simulink library "Memory_Blocks_Lib"  (Simulink 8.7)
settings: Solver=ode45  StartTime=0.0  StopTime=10.0  RelTol=1e-3
libraries: Memory_Blocks_Lib x72, simulink_extras x26, Decoders_Lib x7, Bit_Multiplexers_Lib x5, Byte_Multiplexers_Lib x2, Word_Multiplexers_Lib x1, commutil2 x1
(part 1 of 2)
settings Model: Creator=uzivatel  LastModifiedBy=Jozko Mrkvicka

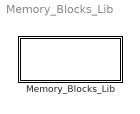
== system Memory_Blocks_Lib ==
  Memory_Blocks_Lib : Subsystem

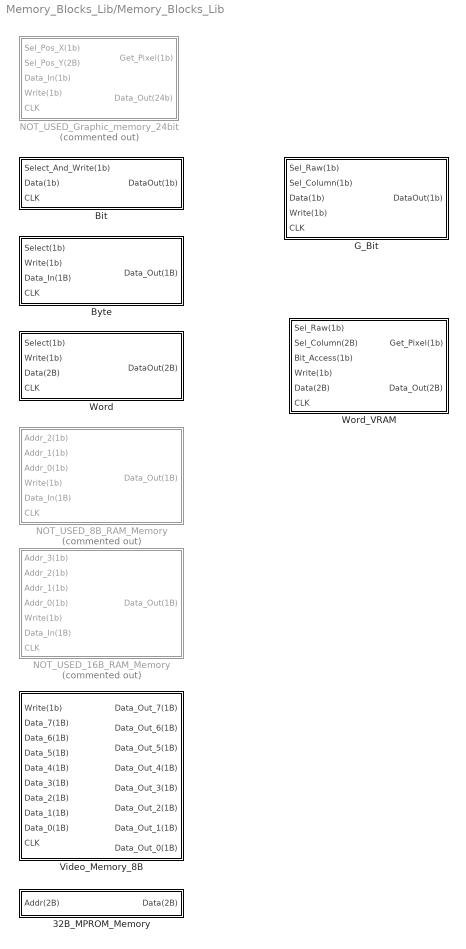
== system Memory_Blocks_Lib/Memory_Blocks_Lib ==
  32B_MPROM_Memory : Subsystem
  Bit : Subsystem
  Byte : Subsystem
  G_Bit : Subsystem
  NOT_USED_16B_RAM_Memory : Subsystem  Commented=on
  NOT_USED_8B_RAM_Memory : Subsystem  Commented=on
  NOT_USED_Graphic_memory_24bit : Subsystem  Commented=on
  Video_Memory_8B : Subsystem
  Word : Subsystem
  Word_VRAM : Subsystem

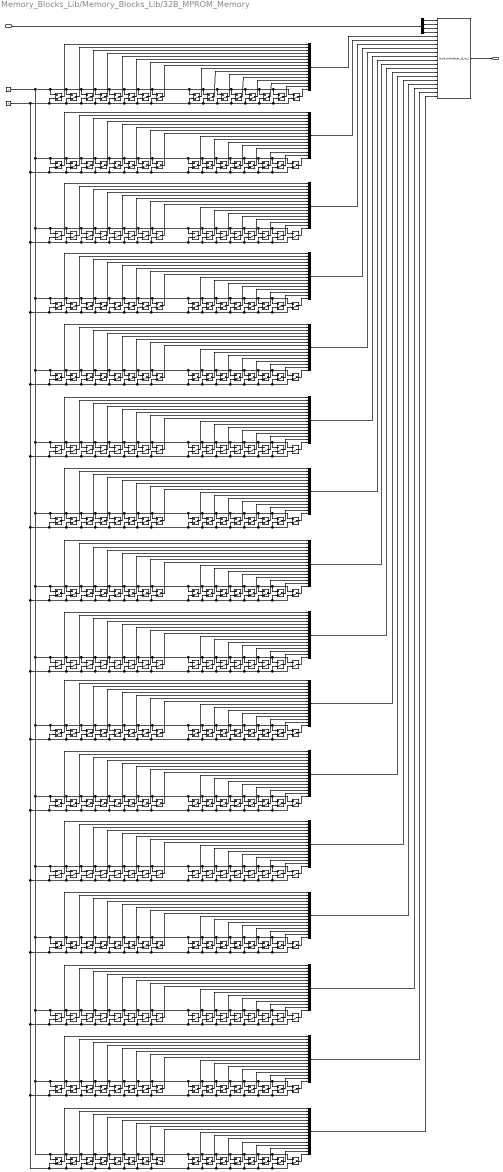
== system Memory_Blocks_Lib/Memory_Blocks_Lib/32B_MPROM_Memory ==
  note: Manually Programmable Read Only Memory (MPROM)
  Addr(2B) : Inport
  Bus Creator{,1..15} (16 alike) : BusCreator  Inputs=16
  Bus Selector : BusSelector  OutputSignals=signal13,signal14,signal15,signal16
  Constant : Constant
  Constant1 : Constant  Value=0
  Manual Switch{,1..156,158..255} (255 alike) : ManualSwitch  CurrentSetting=0
  Manual Switch157 : ManualSwitch
  Word_Multiplexer_16_to_1 : Word_Multiplexers_Lib/Word_Multiplexers_Lib/Word_Multiplexer_16_to_1
  Data(2B) : Outport
  wires:
  Addr(2B)/1 -> Bus Selector/1
  Manual Switch54/1 -> Bus Creator3/16
  Manual Switch59/1 -> Bus Creator3/7
  Manual Switch50/1 -> Bus Creator3/12
  Manual Switch57/1 -> Bus Creator3/5
  Manual Switch53/1 -> Bus Creator3/15
  Manual Switch48/1 -> Bus Creator3/1
  Manual Switch61/1 -> Bus Creator3/9
  Manual Switch52/1 -> Bus Creator3/14
  Manual Switch51/1 -> Bus Creator3/13
  Manual Switch56/1 -> Bus Creator3/4
  Manual Switch49/1 -> Bus Creator3/3
  Manual Switch58/1 -> Bus Creator3/6
  Manual Switch63/1 -> Bus Creator3/11
  Manual Switch62/1 -> Bus Creator3/10
  Manual Switch60/1 -> Bus Creator3/8
  Manual Switch55/1 -> Bus Creator3/2
  Manual Switch14/1 -> Bus Creator/16
  Manual Switch4/1 -> Bus Creator/6
  Manual Switch5/1 -> Bus Creator/7
  Manual Switch3/1 -> Bus Creator/5
  Manual Switch/1 -> Bus Creator/1
  Manual Switch99/1 -> Bus Creator6/13
  Manual Switch98/1 -> Bus Creator6/12
  Manual Switch111/1 -> Bus Creator6/11
  Manual Switch100/1 -> Bus Creator6/14
  Manual Switch110/1 -> Bus Creator6/10
  Manual Switch108/1 -> Bus Creator6/8
  Manual Switch109/1 -> Bus Creator6/9
  Manual Switch102/1 -> Bus Creator6/16
  Manual Switch101/1 -> Bus Creator6/15
  Manual Switch107/1 -> Bus Creator6/7
  Manual Switch104/1 -> Bus Creator6/4
  Manual Switch97/1 -> Bus Creator6/3
  Manual Switch103/1 -> Bus Creator6/2
  Manual Switch96/1 -> Bus Creator6/1
  Manual Switch105/1 -> Bus Creator6/5
  Manual Switch106/1 -> Bus Creator6/6
  Manual Switch85/1 -> Bus Creator5/15
  Manual Switch83/1 -> Bus Creator5/13
  Manual Switch82/1 -> Bus Creator5/12
  Manual Switch86/1 -> Bus Creator5/16
  Manual Switch84/1 -> Bus Creator5/14
  Manual Switch93/1 -> Bus Creator5/9
  Manual Switch91/1 -> Bus Creator5/7
  Manual Switch95/1 -> Bus Creator5/11
  Manual Switch94/1 -> Bus Creator5/10
  Manual Switch92/1 -> Bus Creator5/8
  Manual Switch90/1 -> Bus Creator5/6
  Manual Switch89/1 -> Bus Creator5/5
  Manual Switch88/1 -> Bus Creator5/4
  Manual Switch81/1 -> Bus Creator5/3
  Manual Switch87/1 -> Bus Creator5/2
  Manual Switch80/1 -> Bus Creator5/1
  Manual Switch130/1 -> Bus Creator8/12
  Manual Switch245/1 -> Bus Creator8/11
  Manual Switch234/1 -> Bus Creator8/10
  Manual Switch168/1 -> Bus Creator8/4
  Manual Switch141/1 -> Bus Creator8/13
  Manual Switch128/1 -> Bus Creator8/1
  Manual Switch169/1 -> Bus Creator9/14
  Manual Switch167/1 -> Bus Creator9/13
  Manual Switch166/1 -> Bus Creator9/12
  Manual Switch129/1 -> Bus Creator8/3
  Manual Switch170/1 -> Bus Creator9/15
  Manual Switch162/1 -> Bus Creator8/16
  Manual Switch161/1 -> Bus Creator8/15
  Manual Switch163/1 -> Bus Creator8/2
  Manual Switch171/1 -> Bus Creator9/16
  Manual Switch179/1 -> Bus Creator8/5
  Manual Switch223/1 -> Bus Creator8/9
  Manual Switch212/1 -> Bus Creator8/8
  Manual Switch201/1 -> Bus Creator8/7
  Manual Switch152/1 -> Bus Creator8/14
  Manual Switch190/1 -> Bus Creator8/6
  Manual Switch186/1 -> Bus Creator10/14
  Manual Switch184/1 -> Bus Creator10/12
  Manual Switch197/1 -> Bus Creator10/10
  Manual Switch192/1 -> Bus Creator10/5
  Manual Switch211/1 -> Bus Creator11/7
  Manual Switch209/1 -> Bus Creator11/5
  Manual Switch187/1 -> Bus Creator10/15
  Manual Switch173/1 -> Bus Creator9/4
  Manual Switch195/1 -> Bus Creator10/8
  Manual Switch200/1 -> Bus Creator11/3
  Manual Switch216/1 -> Bus Creator11/11
  Manual Switch199/1 -> Bus Creator11/1
  Manual Switch178/1 -> Bus Creator9/9
  Manual Switch191/1 -> Bus Creator10/4
  Manual Switch214/1 -> Bus Creator11/9
  Manual Switch221/1 -> Bus Creator12/14
  Manual Switch220/1 -> Bus Creator12/13
  Manual Switch232/1 -> Bus Creator12/10
  Manual Switch213/1 -> Bus Creator11/8
  Manual Switch233/1 -> Bus Creator12/11
  Manual Switch231/1 -> Bus Creator12/9
  Manual Switch174/1 -> Bus Creator9/5
  Manual Switch177/1 -> Bus Creator9/8
  Manual Switch189/1 -> Bus Creator10/2
  Manual Switch180/1 -> Bus Creator9/10
  Manual Switch182/1 -> Bus Creator10/1
  Manual Switch203/1 -> Bus Creator11/13
  Manual Switch204/1 -> Bus Creator11/14
  Manual Switch205/1 -> Bus Creator11/15
  Manual Switch181/1 -> Bus Creator9/11
  Manual Switch196/1 -> Bus Creator10/9
  Manual Switch207/1 -> Bus Creator11/2
  Manual Switch222/1 -> Bus Creator12/15
  Manual Switch219/1 -> Bus Creator12/12
  Manual Switch230/1 -> Bus Creator12/8
  Manual Switch198/1 -> Bus Creator10/11
  Manual Switch183/1 -> Bus Creator10/3
  Manual Switch208/1 -> Bus Creator11/4
  Manual Switch194/1 -> Bus Creator10/7
  Manual Switch165/1 -> Bus Creator9/3
  Manual Switch172/1 -> Bus Creator9/2
  Manual Switch229/1 -> Bus Creator12/7
  Manual Switch228/1 -> Bus Creator12/6
  Manual Switch227/1 -> Bus Creator12/5
  Manual Switch202/1 -> Bus Creator11/12
  Manual Switch175/1 -> Bus Creator9/6
  Manual Switch185/1 -> Bus Creator10/13
  Manual Switch215/1 -> Bus Creator11/10
  Manual Switch164/1 -> Bus Creator9/1
  Manual Switch188/1 -> Bus Creator10/16
  Manual Switch210/1 -> Bus Creator11/6
  Manual Switch193/1 -> Bus Creator10/6
  Manual Switch224/1 -> Bus Creator12/16
  Manual Switch206/1 -> Bus Creator11/16
  Manual Switch176/1 -> Bus Creator9/7
  Manual Switch143/1 -> Bus Creator14/11
  Manual Switch236/1 -> Bus Creator13/3
  Manual Switch153/1 -> Bus Creator15/4
  Manual Switch132/1 -> Bus Creator14/15
  Manual Switch140/1 -> Bus Creator14/9
  Manual Switch252/1 -> Bus Creator14/1
  Manual Switch240/1 -> Bus Creator13/15
  Constant/1 -> Manual Switch17/1, Manual Switch24/1, Manual Switch22/1, Manual Switch21/1, Manual Switch20/1, Manual Switch19/1, Manual Switch18/1, Manual Switch31/1, Manual Switch30/1, Manual Switch29/1, Manual Switch28/1, Manual Switch27/1, Manual Switch26/1, Manual Switch25/1, Manual Switch23/1, Manual Switch16/1, Manual Switch33/1, Manual Switch40/1, Manual Switch38/1, Manual Switch37/1, Manual Switch36/1, Manual Switch35/1, Manual Switch34/1, Manual Switch47/1, Manual Switch46/1, Manual Switch45/1, Manual Switch44/1, Manual Switch43/1, Manual Switch42/1, Manual Switch41/1, Manual Switch39/1, Manual Switch32/1, Manual Switch49/1, Manual Switch56/1, Manual Switch54/1, Manual Switch53/1, Manual Switch52/1, Manual Switch51/1, Manual Switch50/1, Manual Switch63/1, Manual Switch62/1, Manual Switch61/1, Manual Switch60/1, Manual Switch59/1, Manual Switch58/1, Manual Switch57/1, Manual Switch55/1, Manual Switch48/1, Manual Switch65/1, Manual Switch72/1, Manual Switch70/1, Manual Switch69/1, Manual Switch68/1, Manual Switch67/1, Manual Switch66/1, Manual Switch79/1, Manual Switch78/1, Manual Switch77/1, Manual Switch76/1, Manual Switch75/1, Manual Switch74/1, Manual Switch73/1, Manual Switch71/1, Manual Switch64/1, Manual Switch81/1, Manual Switch88/1, Manual Switch86/1, Manual Switch85/1, Manual Switch84/1, Manual Switch83/1, Manual Switch82/1, Manual Switch95/1, Manual Switch94/1, Manual Switch93/1, Manual Switch92/1, Manual Switch91/1, Manual Switch90/1, Manual Switch89/1, Manual Switch87/1, Manual Switch80/1, Manual Switch97/1, Manual Switch104/1, Manual Switch102/1, Manual Switch101/1, Manual Switch100/1, Manual Switch99/1, Manual Switch98/1, Manual Switch111/1, Manual Switch110/1, Manual Switch109/1, Manual Switch108/1, Manual Switch107/1, Manual Switch106/1, Manual Switch105/1, Manual Switch103/1, Manual Switch96/1, Manual Switch113/1, Manual Switch120/1, Manual Switch118/1, Manual Switch117/1, Manual Switch116/1, Manual Switch115/1, Manual Switch114/1, Manual Switch127/1, Manual Switch126/1, Manual Switch125/1, Manual Switch124/1, Manual Switch123/1, Manual Switch122/1, Manual Switch121/1, Manual Switch119/1, Manual Switch112/1, Manual Switch129/1, Manual Switch168/1, Manual Switch162/1, Manual Switch161/1, Manual Switch152/1, Manual Switch141/1, Manual Switch130/1, Manual Switch245/1, Manual Switch234/1, Manual Switch223/1, Manual Switch212/1, Manual Switch201/1, Manual Switch190/1, Manual Switch179/1, Manual Switch163/1, Manual Switch128/1, Manual Switch165/1, Manual Switch173/1, Manual Switch171/1, Manual Switch170/1, Manual Switch169/1, Manual Switch167/1, Manual Switch166/1, Manual Switch181/1, Manual Switch180/1, Manual Switch178/1, Manual Switch177/1, Manual Switch176/1, Manual Switch175/1, Manual Switch174/1, Manual Switch172/1, Manual Switch164/1, Manual Switch183/1, Manual Switch191/1, Manual Switch188/1, Manual Switch187/1, Manual Switch186/1, Manual Switch185/1, Manual Switch184/1, Manual Switch198/1, Manual Switch197/1, Manual Switch196/1, Manual Switch195/1, Manual Switch194/1, Manual Switch193/1, Manual Switch192/1, Manual Switch189/1, Manual Switch182/1, Manual Switch200/1, Manual Switch208/1, Manual Switch206/1, Manual Switch205/1, Manual Switch204/1, Manual Switch203/1, Manual Switch202/1, Manual Switch216/1, Manual Switch215/1, Manual Switch214/1, Manual Switch213/1, Manual Switch211/1, Manual Switch210/1, Manual Switch209/1, Manual Switch207/1, Manual Switch199/1, Manual Switch218/1, Manual Switch226/1, Manual Switch224/1, Manual Switch222/1, Manual Switch221/1, Manual Switch220/1, Manual Switch219/1, Manual Switch233/1, Manual Switch232/1, Manual Switch231/1, Manual Switch230/1, Manual Switch229/1, Manual Switch228/1, Manual Switch227/1, Manual Switch225/1, Manual Switch217/1, Manual Switch236/1, Manual Switch243/1, Manual Switch241/1, Manual Switch240/1, Manual Switch239/1, Manual Switch238/1, Manual Switch237/1, Manual Switch251/1, Manual Switch250/1, Manual Switch249/1, Manual Switch248/1, Manual Switch247/1, Manual Switch246/1, Manual Switch244/1, Manual Switch242/1, Manual Switch235/1, Manual Switch253/1, Manual Switch135/1, Manual Switch133/1, Manual Switch132/1, Manual Switch131/1, Manual Switch255/1, Manual Switch254/1, Manual Switch143/1, Manual Switch142/1, Manual Switch140/1, Manual Switch139/1, Manual Switch138/1, Manual Switch137/1, Manual Switch136/1, Manual Switch134/1, Manual Switch252/1, Manual Switch145/1, Manual Switch153/1, Manual Switch150/1, Manual Switch149/1, Manual Switch148/1, Manual Switch147/1, Manual Switch146/1, Manual Switch160/1, Manual Switch159/1, Manual Switch158/1, Manual Switch157/1, Manual Switch156/1, Manual Switch155/1, Manual Switch154/1, Manual Switch151/1, Manual Switch144/1, Manual Switch1/1, Manual Switch2/1, Manual Switch14/1, Manual Switch13/1, Manual Switch12/1, Manual Switch11/1, Manual Switch10/1, Manual Switch9/1, Manual Switch8/1, Manual Switch7/1, Manual Switch6/1, Manual Switch5/1, Manual Switch4/1, Manual Switch3/1, Manual Switch15/1, Manual Switch/1
  Manual Switch254/1 -> Bus Creator14/12
  Manual Switch159/1 -> Bus Creator15/10
  Manual Switch145/1 -> Bus Creator15/3
  Manual Switch151/1 -> Bus Creator15/2
  Manual Switch144/1 -> Bus Creator15/1
  Manual Switch139/1 -> Bus Creator14/8
  Manual Switch138/1 -> Bus Creator14/7
  Manual Switch134/1 -> Bus Creator14/2
  Manual Switch242/1 -> Bus Creator13/2
  Manual Switch239/1 -> Bus Creator13/14
  Manual Switch253/1 -> Bus Creator14/3
  Manual Switch251/1 -> Bus Creator13/11
  Manual Switch149/1 -> Bus Creator15/15
  Manual Switch217/1 -> Bus Creator12/1
  Manual Switch255/1 -> Bus Creator14/13
  Manual Switch249/1 -> Bus Creator13/9
  Manual Switch235/1 -> Bus Creator13/1
  Manual Switch131/1 -> Bus Creator14/14
  Manual Switch225/1 -> Bus Creator12/2
  Manual Switch218/1 -> Bus Creator12/3
  Manual Switch248/1 -> Bus Creator13/8
  Manual Switch136/1 -> Bus Creator14/5
  Manual Switch135/1 -> Bus Creator14/4
  Manual Switch147/1 -> Bus Creator15/13
  Manual Switch146/1 -> Bus Creator15/12
  Manual Switch237/1 -> Bus Creator13/12
  Manual Switch243/1 -> Bus Creator13/4
  Manual Switch250/1 -> Bus Creator13/10
  Manual Switch142/1 -> Bus Creator14/10
  Manual Switch148/1 -> Bus Creator15/14
  Manual Switch160/1 -> Bus Creator15/11
  Manual Switch238/1 -> Bus Creator13/13
  Manual Switch137/1 -> Bus Creator14/6
  Manual Switch158/1 -> Bus Creator15/9
  Manual Switch246/1 -> Bus Creator13/6
  Manual Switch247/1 -> Bus Creator13/7
  Manual Switch157/1 -> Bus Creator15/8
  Manual Switch244/1 -> Bus Creator13/5
  Manual Switch133/1 -> Bus Creator14/16
  Manual Switch150/1 -> Bus Creator15/16
  Manual Switch156/1 -> Bus Creator15/7
  Manual Switch155/1 -> Bus Creator15/6
  Manual Switch154/1 -> Bus Creator15/5
  Manual Switch226/1 -> Bus Creator12/4
  Manual Switch241/1 -> Bus Creator13/16
  Manual Switch13/1 -> Bus Creator/15
  Manual Switch6/1 -> Bus Creator/8
  Manual Switch11/1 -> Bus Creator/13
  Manual Switch9/1 -> Bus Creator/11
  Manual Switch15/1 -> Bus Creator/2
  Manual Switch8/1 -> Bus Creator/10
  Manual Switch10/1 -> Bus Creator/12
  Manual Switch33/1 -> Bus Creator2/3
  Manual Switch35/1 -> Bus Creator2/13
  Manual Switch44/1 -> Bus Creator2/8
  Manual Switch40/1 -> Bus Creator2/4
  Manual Switch43/1 -> Bus Creator2/7
  Manual Switch39/1 -> Bus Creator2/2
  Manual Switch36/1 -> Bus Creator2/14
  Manual Switch47/1 -> Bus Creator2/11
  Manual Switch41/1 -> Bus Creator2/5
  Manual Switch38/1 -> Bus Creator2/16
  Manual Switch34/1 -> Bus Creator2/12
  Manual Switch45/1 -> Bus Creator2/9
  Manual Switch32/1 -> Bus Creator2/1
  Manual Switch42/1 -> Bus Creator2/6
  Manual Switch46/1 -> Bus Creator2/10
  Manual Switch37/1 -> Bus Creator2/15
  Bus Creator2/1 -> Word_Multiplexer_16_to_1/7
  Bus Creator1/1 -> Word_Multiplexer_16_to_1/6
  Bus Creator5/1 -> Word_Multiplexer_16_to_1/10
  Bus Selector/1 -> Word_Multiplexer_16_to_1/1  "<signal13>"
  Bus Creator15/1 -> Word_Multiplexer_16_to_1/20
  Bus Selector/4 -> Word_Multiplexer_16_to_1/4  "<signal16>"
  Bus Creator11/1 -> Word_Multiplexer_16_to_1/16
  Bus Creator14/1 -> Word_Multiplexer_16_to_1/19
  Bus Creator/1 -> Word_Multiplexer_16_to_1/5
  Bus Creator9/1 -> Word_Multiplexer_16_to_1/14
  Bus Creator12/1 -> Word_Multiplexer_16_to_1/17
  Bus Creator13/1 -> Word_Multiplexer_16_to_1/18
  Bus Selector/2 -> Word_Multiplexer_16_to_1/2  "<signal14>"
  Bus Creator4/1 -> Word_Multiplexer_16_to_1/9
  Bus Creator6/1 -> Word_Multiplexer_16_to_1/11
  Bus Selector/3 -> Word_Multiplexer_16_to_1/3  "<signal15>"
  Bus Creator3/1 -> Word_Multiplexer_16_to_1/8
  Bus Creator8/1 -> Word_Multiplexer_16_to_1/13
  Bus Creator10/1 -> Word_Multiplexer_16_to_1/15
  Word_Multiplexer_16_to_1/1 -> Data(2B)/1
  Bus Creator7/1 -> Word_Multiplexer_16_to_1/12
  Manual Switch70/1 -> Bus Creator4/16
  Manual Switch69/1 -> Bus Creator4/15
  Manual Switch79/1 -> Bus Creator4/11
  Manual Switch75/1 -> Bus Creator4/7
  Manual Switch73/1 -> Bus Creator4/5
  Manual Switch68/1 -> Bus Creator4/14
  Manual Switch65/1 -> Bus Creator4/3
  Manual Switch71/1 -> Bus Creator4/2
  Manual Switch74/1 -> Bus Creator4/6
  Manual Switch76/1 -> Bus Creator4/8
  Manual Switch64/1 -> Bus Creator4/1
  Manual Switch72/1 -> Bus Creator4/4
  Manual Switch78/1 -> Bus Creator4/10
  Manual Switch66/1 -> Bus Creator4/12
  Manual Switch77/1 -> Bus Creator4/9
  Manual Switch67/1 -> Bus Creator4/13
  Manual Switch127/1 -> Bus Creator7/11
  Manual Switch125/1 -> Bus Creator7/9
  Manual Switch119/1 -> Bus Creator7/2
  Manual Switch122/1 -> Bus Creator7/6
  Manual Switch112/1 -> Bus Creator7/1
  Manual Switch121/1 -> Bus Creator7/5
  Manual Switch120/1 -> Bus Creator7/4
  Manual Switch113/1 -> Bus Creator7/3
  Manual Switch124/1 -> Bus Creator7/8
  Manual Switch126/1 -> Bus Creator7/10
  Manual Switch123/1 -> Bus Creator7/7
  Manual Switch2/1 -> Bus Creator/4
  Manual Switch12/1 -> Bus Creator/14
  Manual Switch115/1 -> Bus Creator7/13
  Manual Switch114/1 -> Bus Creator7/12
  Manual Switch7/1 -> Bus Creator/9
  Manual Switch1/1 -> Bus Creator/3
  Manual Switch118/1 -> Bus Creator7/16
  Manual Switch116/1 -> Bus Creator7/14
  Manual Switch117/1 -> Bus Creator7/15
  Manual Switch24/1 -> Bus Creator1/4
  Manual Switch22/1 -> Bus Creator1/16
  Manual Switch30/1 -> Bus Creator1/10
  Manual Switch26/1 -> Bus Creator1/6
  Manual Switch20/1 -> Bus Creator1/14
  Manual Switch19/1 -> Bus Creator1/13
  Constant1/1 -> Manual Switch23/2, Manual Switch17/2, Manual Switch25/2, Manual Switch26/2, Manual Switch22/2, Manual Switch21/2, Manual Switch20/2, Manual Switch19/2, Manual Switch18/2, Manual Switch31/2, Manual Switch30/2, Manual Switch29/2, Manual Switch28/2, Manual Switch27/2, Manual Switch24/2, Manual Switch16/2, Manual Switch39/2, Manual Switch33/2, Manual Switch41/2, Manual Switch42/2, Manual Switch38/2, Manual Switch37/2, Manual Switch36/2, Manual Switch35/2, Manual Switch34/2, Manual Switch47/2, Manual Switch46/2, Manual Switch45/2, Manual Switch44/2, Manual Switch43/2, Manual Switch40/2, Manual Switch32/2, Manual Switch55/2, Manual Switch49/2, Manual Switch57/2, Manual Switch58/2, Manual Switch54/2, Manual Switch53/2, Manual Switch52/2, Manual Switch51/2, Manual Switch50/2, Manual Switch63/2, Manual Switch62/2, Manual Switch61/2, Manual Switch60/2, Manual Switch59/2, Manual Switch56/2, Manual Switch48/2, Manual Switch71/2, Manual Switch65/2, Manual Switch73/2, Manual Switch74/2, Manual Switch70/2, Manual Switch69/2, Manual Switch68/2, Manual Switch67/2, Manual Switch66/2, Manual Switch79/2, Manual Switch78/2, Manual Switch77/2, Manual Switch76/2, Manual Switch75/2, Manual Switch72/2, Manual Switch64/2, Manual Switch103/2, Manual Switch97/2, Manual Switch105/2, Manual Switch106/2, Manual Switch102/2, Manual Switch101/2, Manual Switch100/2, Manual Switch99/2, Manual Switch98/2, Manual Switch111/2, Manual Switch110/2, Manual Switch109/2, Manual Switch108/2, Manual Switch107/2, Manual Switch104/2, Manual Switch96/2, Manual Switch119/2, Manual Switch113/2, Manual Switch121/2, Manual Switch122/2, Manual Switch118/2, Manual Switch117/2, Manual Switch116/2, Manual Switch115/2, Manual Switch114/2, Manual Switch127/2, Manual Switch126/2, Manual Switch125/2, Manual Switch124/2, Manual Switch123/2, Manual Switch120/2, Manual Switch112/2, Manual Switch163/2, Manual Switch129/2, Manual Switch179/2, Manual Switch190/2, Manual Switch162/2, Manual Switch161/2, Manual Switch152/2, Manual Switch141/2, Manual Switch130/2, Manual Switch245/2, Manual Switch234/2, Manual Switch223/2, Manual Switch212/2, Manual Switch201/2, Manual Switch168/2, Manual Switch128/2, Manual Switch172/2, Manual Switch165/2, Manual Switch174/2, Manual Switch175/2, Manual Switch171/2, Manual Switch170/2, Manual Switch169/2, Manual Switch167/2, Manual Switch166/2, Manual Switch181/2, Manual Switch180/2, Manual Switch178/2, Manual Switch177/2, Manual Switch176/2, Manual Switch173/2, Manual Switch164/2, Manual Switch189/2, Manual Switch183/2, Manual Switch192/2, Manual Switch193/2, Manual Switch188/2, Manual Switch187/2, Manual Switch186/2, Manual Switch185/2, Manual Switch184/2, Manual Switch198/2, Manual Switch197/2, Manual Switch196/2, Manual Switch195/2, Manual Switch194/2, Manual Switch191/2, Manual Switch182/2, Manual Switch207/2, Manual Switch200/2, Manual Switch209/2, Manual Switch210/2, Manual Switch206/2, Manual Switch205/2, Manual Switch204/2, Manual Switch203/2, Manual Switch202/2, Manual Switch216/2, Manual Switch215/2, Manual Switch214/2, Manual Switch213/2, Manual Switch211/2, Manual Switch208/2, Manual Switch199/2, Manual Switch225/2, Manual Switch218/2, Manual Switch227/2, Manual Switch228/2, Manual Switch224/2, Manual Switch222/2, Manual Switch221/2, Manual Switch220/2, Manual Switch219/2, Manual Switch233/2, Manual Switch232/2, Manual Switch231/2, Manual Switch230/2, Manual Switch229/2, Manual Switch226/2, Manual Switch217/2, Manual Switch242/2, Manual Switch236/2, Manual Switch244/2, Manual Switch246/2, Manual Switch241/2, Manual Switch240/2, Manual Switch239/2, Manual Switch238/2, Manual Switch237/2, Manual Switch251/2, Manual Switch250/2, Manual Switch249/2, Manual Switch248/2, Manual Switch247/2, Manual Switch243/2, Manual Switch235/2, Manual Switch134/2, Manual Switch253/2, Manual Switch136/2, Manual Switch137/2, Manual Switch133/2, Manual Switch132/2, Manual Switch131/2, Manual Switch255/2, Manual Switch254/2, Manual Switch143/2, Manual Switch142/2, Manual Switch140/2, Manual Switch139/2, Manual Switch138/2, Manual Switch135/2, Manual Switch252/2, Manual Switch151/2, Manual Switch145/2, Manual Switch154/2, Manual Switch155/2, Manual Switch150/2, Manual Switch149/2, Manual Switch148/2, Manual Switch147/2, Manual Switch146/2, Manual Switch160/2, Manual Switch159/2, Manual Switch158/2, Manual Switch157/2, Manual Switch156/2, Manual Switch153/2, Manual Switch144/2, Manual Switch87/2, Manual Switch81/2, Manual Switch89/2, Manual Switch90/2, Manual Switch86/2, Manual Switch85/2, Manual Switch84/2, Manual Switch83/2, Manual Switch82/2, Manual Switch95/2, Manual Switch94/2, Manual Switch93/2, Manual Switch92/2, Manual Switch91/2, Manual Switch88/2, Manual Switch80/2, Manual Switch15/2, Manual Switch1/2, Manual Switch3/2, Manual Switch4/2, Manual Switch14/2, Manual Switch13/2, Manual Switch12/2, Manual Switch11/2, Manual Switch10/2, Manual Switch9/2, Manual Switch8/2, Manual Switch7/2, Manual Switch6/2, Manual Switch5/2, Manual Switch2/2, Manual Switch/2
  Manual Switch27/1 -> Bus Creator1/7
  Manual Switch21/1 -> Bus Creator1/15
  Manual Switch25/1 -> Bus Creator1/5
  Manual Switch17/1 -> Bus Creator1/3
  Manual Switch31/1 -> Bus Creator1/11
  Manual Switch29/1 -> Bus Creator1/9
  Manual Switch28/1 -> Bus Creator1/8
  Manual Switch23/1 -> Bus Creator1/2
  Manual Switch16/1 -> Bus Creator1/1
  Manual Switch18/1 -> Bus Creator1/12

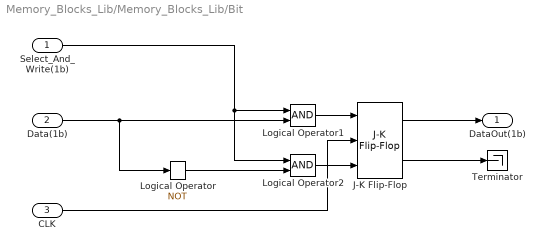
== system Memory_Blocks_Lib/Memory_Blocks_Lib/Bit ==
  Select_And_Write(1b) : Inport  OutDataTypeStr=boolean
  Data(1b) : Inport  Port=2  OutDataTypeStr=boolean
  CLK : Inport  Port=3  OutDataTypeStr=double
  J-K Flip-Flop : simulink_extras/Flip Flops/J-K Flip-Flop  initial_condition=0
  Logical Operator : Logic  Operator=NOT  IconShape=distinctive  AllPortsSameDT=off  OutDataTypeStr=boolean
  Logical Operator1 : Logic  IconShape=distinctive  AllPortsSameDT=off  OutDataTypeStr=boolean
  Logical Operator2 : Logic  IconShape=distinctive  AllPortsSameDT=off  OutDataTypeStr=boolean
  Terminator : Terminator
  DataOut(1b) : Outport
  wires:
  Data(1b)/1 -> Logical Operator/1, Logical Operator1/2
  J-K Flip-Flop/2 -> Terminator/1
  J-K Flip-Flop/1 -> DataOut(1b)/1
  CLK/1 -> J-K Flip-Flop/2
  Select_And_Write(1b)/1 -> Logical Operator2/1, Logical Operator1/1
  Logical Operator/1 -> Logical Operator2/2
  Logical Operator1/1 -> J-K Flip-Flop/1
  Logical Operator2/1 -> J-K Flip-Flop/3

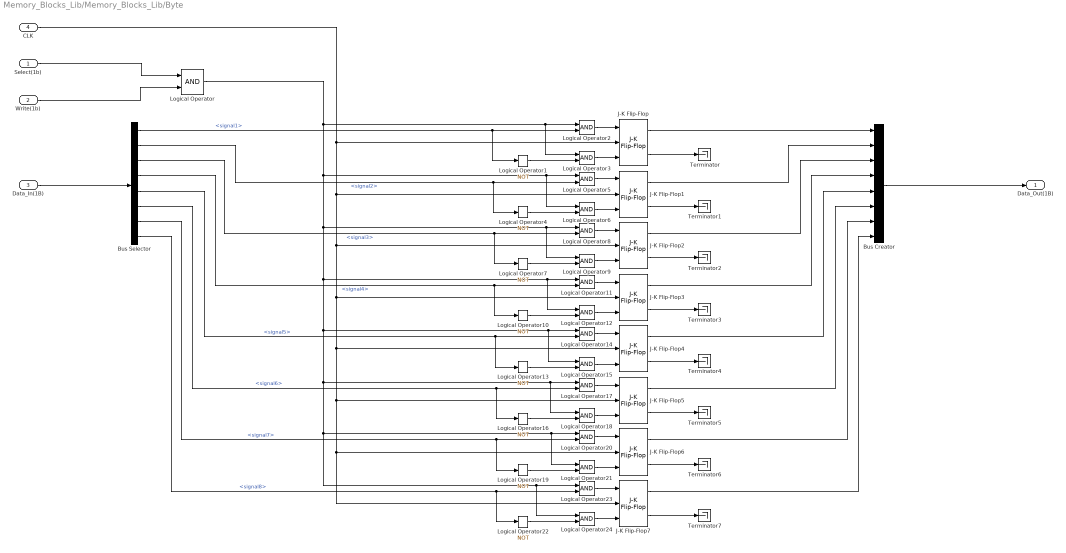
== system Memory_Blocks_Lib/Memory_Blocks_Lib/Byte ==
  Select(1b) : Inport
  Write(1b) : Inport  Port=2
  Data_In(1B) : Inport  Port=3
  CLK : Inport  Port=4  OutDataTypeStr=double
  Bus Creator : BusCreator  Inputs=8
  Bus Selector : BusSelector  OutputSignals=signal1,signal2,signal3,signal4,signal5,signal6,signal7,signal8
  J-K Flip-Flop{,1..7} (8 alike) : simulink_extras/Flip Flops/J-K Flip-Flop  initial_condition=0
  Logical Operator{,2..3,5..6,8..9,11..12,14..15,17..18,20..21,23..24} (17 alike) : Logic  IconShape=distinctive  AllPortsSameDT=off  OutDataTypeStr=boolean
  Logical Operator{1,4,7,10,13,16,19,22} (8 alike) : Logic  Operator=NOT  IconShape=distinctive  AllPortsSameDT=off  OutDataTypeStr=boolean
  Terminator{,1..7} (8 alike) : Terminator
  Data_Out(1B) : Outport
  wires:
  Write(1b)/1 -> Logical Operator/2
  Select(1b)/1 -> Logical Operator/1
  Data_In(1B)/1 -> Bus Selector/1
  J-K Flip-Flop7/1 -> Bus Creator/8
  J-K Flip-Flop6/1 -> Bus Creator/7
  J-K Flip-Flop5/1 -> Bus Creator/6
  J-K Flip-Flop4/1 -> Bus Creator/5
  J-K Flip-Flop3/1 -> Bus Creator/4
  J-K Flip-Flop2/1 -> Bus Creator/3
  J-K Flip-Flop1/1 -> Bus Creator/2
  J-K Flip-Flop/1 -> Bus Creator/1
  Bus Selector/1 -> Logical Operator1/1, Logical Operator2/2  "<signal1>"
  J-K Flip-Flop/2 -> Terminator/1
  Logical Operator1/1 -> Logical Operator3/2
  Logical Operator2/1 -> J-K Flip-Flop/1
  Logical Operator3/1 -> J-K Flip-Flop/3
  Bus Selector/2 -> Logical Operator4/1, Logical Operator5/2  "<signal2>"
  J-K Flip-Flop1/2 -> Terminator1/1
  Logical Operator4/1 -> Logical Operator6/2
  Logical Operator5/1 -> J-K Flip-Flop1/1
  Logical Operator6/1 -> J-K Flip-Flop1/3
  Bus Selector/3 -> Logical Operator7/1, Logical Operator8/2  "<signal3>"
  J-K Flip-Flop2/2 -> Terminator2/1
  Logical Operator7/1 -> Logical Operator9/2
  Logical Operator8/1 -> J-K Flip-Flop2/1
  Logical Operator9/1 -> J-K Flip-Flop2/3
  Bus Selector/4 -> Logical Operator11/2, Logical Operator10/1  "<signal4>"
  J-K Flip-Flop3/2 -> Terminator3/1
  Logical Operator10/1 -> Logical Operator12/2
  Logical Operator11/1 -> J-K Flip-Flop3/1
  Logical Operator12/1 -> J-K Flip-Flop3/3
  Bus Selector/5 -> Logical Operator14/2, Logical Operator13/1  "<signal5>"
  J-K Flip-Flop4/2 -> Terminator4/1
  Logical Operator13/1 -> Logical Operator15/2
  Logical Operator14/1 -> J-K Flip-Flop4/1
  Logical Operator15/1 -> J-K Flip-Flop4/3
  Bus Selector/6 -> Logical Operator17/2, Logical Operator16/1  "<signal6>"
  J-K Flip-Flop5/2 -> Terminator5/1
  Logical Operator16/1 -> Logical Operator18/2
  Logical Operator17/1 -> J-K Flip-Flop5/1
  Logical Operator18/1 -> J-K Flip-Flop5/3
  Bus Selector/7 -> Logical Operator19/1, Logical Operator20/2  "<signal7>"
  J-K Flip-Flop6/2 -> Terminator6/1
  Logical Operator19/1 -> Logical Operator21/2
  Logical Operator20/1 -> J-K Flip-Flop6/1
  Logical Operator21/1 -> J-K Flip-Flop6/3
  Bus Selector/8 -> Logical Operator22/1, Logical Operator23/2  "<signal8>"
  J-K Flip-Flop7/2 -> Terminator7/1
  CLK/1 -> J-K Flip-Flop6/2, J-K Flip-Flop7/2, J-K Flip-Flop5/2, J-K Flip-Flop4/2, J-K Flip-Flop3/2, J-K Flip-Flop2/2, J-K Flip-Flop1/2, J-K Flip-Flop/2
  Logical Operator/1 -> Logical Operator24/1, Logical Operator23/1, Logical Operator21/1, Logical Operator20/1, Logical Operator17/1, Logical Operator18/1, Logical Operator15/1, Logical Operator14/1, Logical Operator12/1, Logical Operator11/1, Logical Operator9/1, Logical Operator8/1, Logical Operator6/1, Logical Operator5/1, Logical Operator3/1, Logical Operator2/1
  Logical Operator22/1 -> Logical Operator24/2
  Logical Operator23/1 -> J-K Flip-Flop7/1
  Logical Operator24/1 -> J-K Flip-Flop7/3
  Bus Creator/1 -> Data_Out(1B)/1

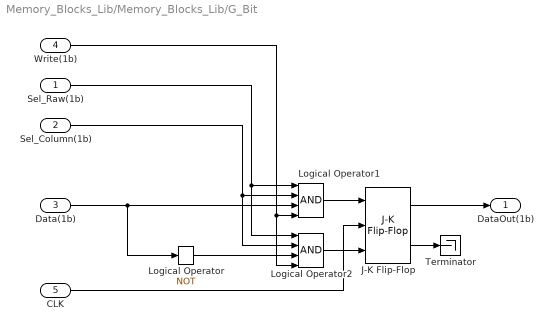
== system Memory_Blocks_Lib/Memory_Blocks_Lib/G_Bit ==
  Sel_Raw(1b) : Inport  OutDataTypeStr=boolean
  Sel_Column(1b) : Inport  Port=2  OutDataTypeStr=boolean
  Data(1b) : Inport  Port=3  OutDataTypeStr=boolean
  Write(1b) : Inport  Port=4  OutDataTypeStr=boolean
  CLK : Inport  Port=5  OutDataTypeStr=double
  J-K Flip-Flop : simulink_extras/Flip Flops/J-K Flip-Flop  initial_condition=0
  Logical Operator : Logic  Operator=NOT  IconShape=distinctive  AllPortsSameDT=off  OutDataTypeStr=boolean
  Logical Operator1 : Logic  Inputs=4  IconShape=distinctive  AllPortsSameDT=off  OutDataTypeStr=boolean
  Logical Operator2 : Logic  Inputs=4  IconShape=distinctive  AllPortsSameDT=off  OutDataTypeStr=boolean
  Terminator : Terminator
  DataOut(1b) : Outport
  wires:
  Logical Operator2/1 -> J-K Flip-Flop/3
  Logical Operator1/1 -> J-K Flip-Flop/1
  Logical Operator/1 -> Logical Operator2/3
  Sel_Column(1b)/1 -> Logical Operator2/2, Logical Operator1/2
  CLK/1 -> J-K Flip-Flop/2
  J-K Flip-Flop/1 -> DataOut(1b)/1
  J-K Flip-Flop/2 -> Terminator/1
  Data(1b)/1 -> Logical Operator1/3, Logical Operator/1
  Sel_Raw(1b)/1 -> Logical Operator2/1, Logical Operator1/1
  Write(1b)/1 -> Logical Operator1/4, Logical Operator2/4

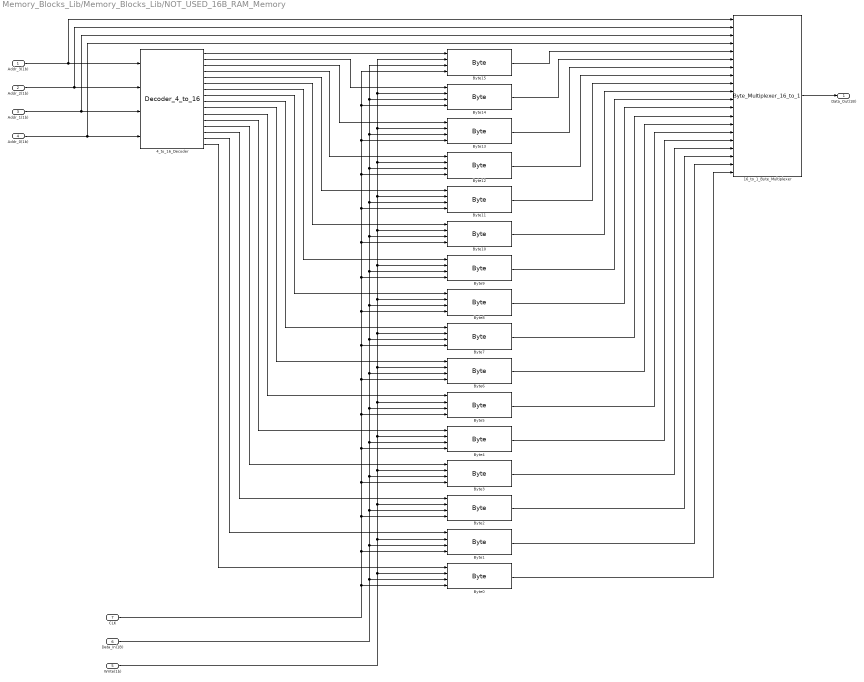
== system Memory_Blocks_Lib/Memory_Blocks_Lib/NOT_USED_16B_RAM_Memory ==
  Addr_3(1b) : Inport
  Addr_2(1b) : Inport  Port=2
  Addr_1(1b) : Inport  Port=3
  Addr_0(1b) : Inport  Port=4
  Write(1b) : Inport  Port=5
  Data_In(1B) : Inport  Port=6
  CLK : Inport  Port=7  OutDataTypeStr=double
  16_to_1_Byte_Multiplexer : Byte_Multiplexers_Lib/Byte_Multiplexers_Lib/Byte_Multiplexer_16_to_1
  4_to_16_Decoder : Decoders_Lib/Decoders_Lib/Decoder_4_to_16
  Byte{0..15} (16 alike) : Memory_Blocks_Lib/Memory_Blocks_Lib/Byte
  Data_Out(1B) : Outport
  wires:
  16_to_1_Byte_Multiplexer/1 -> Data_Out(1B)/1
  Byte0/1 -> 16_to_1_Byte_Multiplexer/20
  Byte1/1 -> 16_to_1_Byte_Multiplexer/19
  Byte2/1 -> 16_to_1_Byte_Multiplexer/18
  Byte3/1 -> 16_to_1_Byte_Multiplexer/17
  Byte4/1 -> 16_to_1_Byte_Multiplexer/16
  Byte5/1 -> 16_to_1_Byte_Multiplexer/15
  Byte6/1 -> 16_to_1_Byte_Multiplexer/14
  Byte7/1 -> 16_to_1_Byte_Multiplexer/13
  Byte8/1 -> 16_to_1_Byte_Multiplexer/12
  Byte9/1 -> 16_to_1_Byte_Multiplexer/11
  Byte10/1 -> 16_to_1_Byte_Multiplexer/10
  Byte11/1 -> 16_to_1_Byte_Multiplexer/9
  Byte12/1 -> 16_to_1_Byte_Multiplexer/8
  Byte13/1 -> 16_to_1_Byte_Multiplexer/7
  Byte14/1 -> 16_to_1_Byte_Multiplexer/6
  Byte15/1 -> 16_to_1_Byte_Multiplexer/5
  4_to_16_Decoder/16 -> Byte0/1
  4_to_16_Decoder/15 -> Byte1/1
  4_to_16_Decoder/14 -> Byte2/1
  4_to_16_Decoder/13 -> Byte3/1
  4_to_16_Decoder/12 -> Byte4/1
  4_to_16_Decoder/11 -> Byte5/1
  4_to_16_Decoder/10 -> Byte6/1
  4_to_16_Decoder/9 -> Byte7/1
  4_to_16_Decoder/8 -> Byte8/1
  4_to_16_Decoder/7 -> Byte9/1
  4_to_16_Decoder/6 -> Byte10/1
  4_to_16_Decoder/5 -> Byte11/1
  4_to_16_Decoder/4 -> Byte12/1
  4_to_16_Decoder/3 -> Byte13/1
  4_to_16_Decoder/2 -> Byte14/1
  Addr_3(1b)/1 -> 4_to_16_Decoder/1, 16_to_1_Byte_Multiplexer/1
  4_to_16_Decoder/1 -> Byte15/1
  Write(1b)/1 -> Byte15/2, Byte14/2, Byte13/2, Byte12/2, Byte11/2, Byte10/2, Byte9/2, Byte8/2, Byte7/2, Byte6/2, Byte5/2, Byte4/2, Byte3/2, Byte2/2, Byte1/2, Byte0/2
  Data_In(1B)/1 -> Byte15/3, Byte14/3, Byte13/3, Byte12/3, Byte11/3, Byte10/3, Byte9/3, Byte8/3, Byte7/3, Byte6/3, Byte5/3, Byte4/3, Byte3/3, Byte2/3, Byte1/3, Byte0/3
  CLK/1 -> Byte15/4, Byte14/4, Byte13/4, Byte12/4, Byte11/4, Byte10/4, Byte9/4, Byte8/4, Byte7/4, Byte6/4, Byte5/4, Byte4/4, Byte3/4, Byte2/4, Byte1/4, Byte0/4
  Addr_2(1b)/1 -> 4_to_16_Decoder/2, 16_to_1_Byte_Multiplexer/2
  Addr_1(1b)/1 -> 4_to_16_Decoder/3, 16_to_1_Byte_Multiplexer/3
  Addr_0(1b)/1 -> 16_to_1_Byte_Multiplexer/4, 4_to_16_Decoder/4

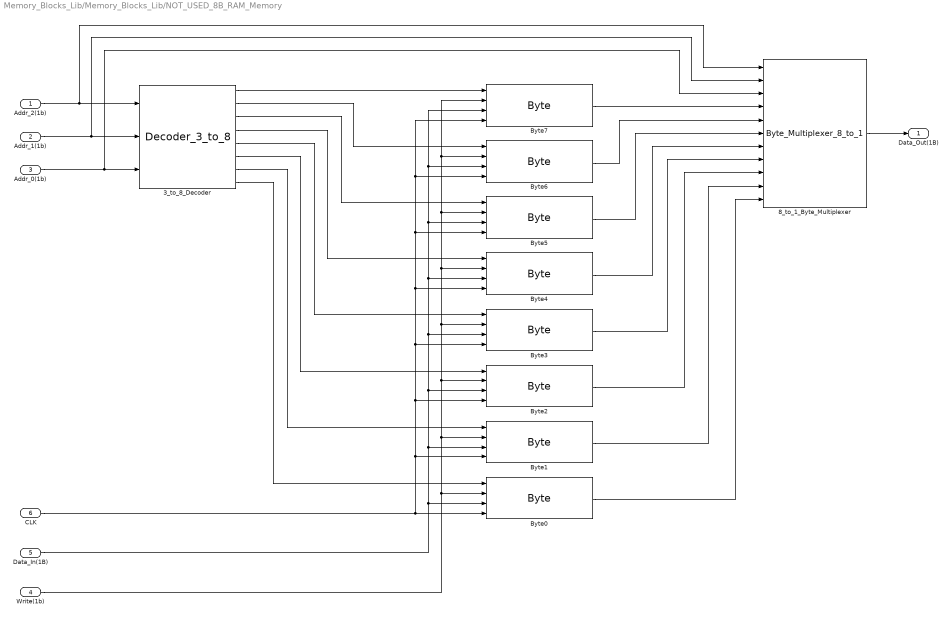
== system Memory_Blocks_Lib/Memory_Blocks_Lib/NOT_USED_8B_RAM_Memory ==
  Addr_2(1b) : Inport
  Addr_1(1b) : Inport  Port=2
  Addr_0(1b) : Inport  Port=3
  Write(1b) : Inport  Port=4
  Data_In(1B) : Inport  Port=5
  CLK : Inport  Port=6  OutDataTypeStr=double
  3_to_8_Decoder : Decoders_Lib/Decoders_Lib/Decoder_3_to_8
  8_to_1_Byte_Multiplexer : Byte_Multiplexers_Lib/Byte_Multiplexers_Lib/Byte_Multiplexer_8_to_1
  Byte{0..7} (8 alike) : Memory_Blocks_Lib/Memory_Blocks_Lib/Byte
  Data_Out(1B) : Outport
  wires:
  8_to_1_Byte_Multiplexer/1 -> Data_Out(1B)/1
  Byte0/1 -> 8_to_1_Byte_Multiplexer/11
  Byte1/1 -> 8_to_1_Byte_Multiplexer/10
  Byte2/1 -> 8_to_1_Byte_Multiplexer/9
  Byte3/1 -> 8_to_1_Byte_Multiplexer/8
  Byte4/1 -> 8_to_1_Byte_Multiplexer/7
  Byte5/1 -> 8_to_1_Byte_Multiplexer/6
  Byte6/1 -> 8_to_1_Byte_Multiplexer/5
  Byte7/1 -> 8_to_1_Byte_Multiplexer/4
  3_to_8_Decoder/8 -> Byte0/1
  3_to_8_Decoder/7 -> Byte1/1
  3_to_8_Decoder/6 -> Byte2/1
  3_to_8_Decoder/5 -> Byte3/1
  3_to_8_Decoder/4 -> Byte4/1
  3_to_8_Decoder/3 -> Byte5/1
  3_to_8_Decoder/2 -> Byte6/1
  3_to_8_Decoder/1 -> Byte7/1
  Write(1b)/1 -> Byte7/2, Byte6/2, Byte5/2, Byte4/2, Byte3/2, Byte2/2, Byte1/2, Byte0/2
  Data_In(1B)/1 -> Byte7/3, Byte6/3, Byte5/3, Byte4/3, Byte3/3, Byte2/3, Byte1/3, Byte0/3
  CLK/1 -> Byte7/4, Byte6/4, Byte5/4, Byte4/4, Byte3/4, Byte2/4, Byte1/4, Byte0/4
  Addr_2(1b)/1 -> 8_to_1_Byte_Multiplexer/1, 3_to_8_Decoder/1
  Addr_1(1b)/1 -> 8_to_1_Byte_Multiplexer/2, 3_to_8_Decoder/2
  Addr_0(1b)/1 -> 8_to_1_Byte_Multiplexer/3, 3_to_8_Decoder/3

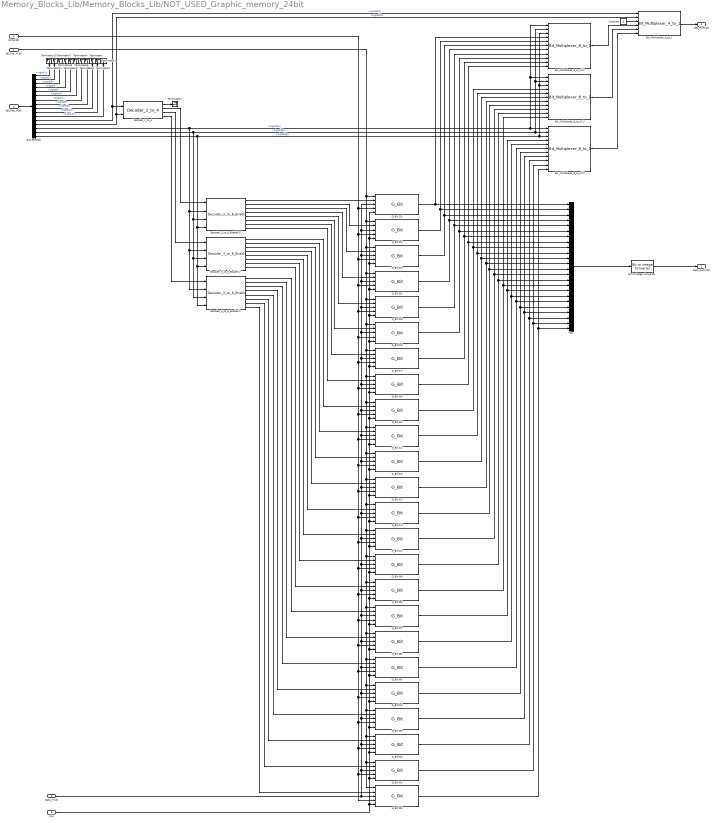
== system Memory_Blocks_Lib/Memory_Blocks_Lib/NOT_USED_Graphic_memory_24bit ==
  Sel_Pos_X(1b) : Inport
  Sel_Pos_Y(2B) : Inport  Port=2
  Data_In(1b) : Inport  Port=3
  Write(1b) : Inport  Port=4
  CLK : Inport  Port=5
  Bit to Integer Converter : commutil2/Bit to Integer Converter  nbits=24  bitOrder=MSB first  signedOutputValues=Unsigned  outDtype=uint32  outDtypeSigned=Inherit via internal rule
  Bit_Multiplexer_4_to_1 : Bit_Multiplexers_Lib/Bit_Multiplexers_Lib/Bit_Multiplexer_4_to_1
  Bit_Multiplexer_8_to_1(0) : Bit_Multiplexers_Lib/Bit_Multiplexers_Lib/Bit_Multiplexer_8_to_1
  Bit_Multiplexer_8_to_1(1) : Bit_Multiplexers_Lib/Bit_Multiplexers_Lib/Bit_Multiplexer_8_to_1
  Bit_Multiplexer_8_to_1(2) : Bit_Multiplexers_Lib/Bit_Multiplexers_Lib/Bit_Multiplexer_8_to_1
  Bus Selector : BusSelector  OutputSignals=signal1,signal2,signal3,signal4,signal5,signal6,signal7,signal8,signal9,signal10,signal11,signal12,signal13,signal14,signal15,signal16
  Constant : Constant  OutDataTypeStr=boolean
  Decoder_2_to_4 : Decoders_Lib/Decoders_Lib/Decoder_2_to_4
  Decoder_3_to_8_Enable(0) : Decoders_Lib/Decoders_Lib/Decoder_3_to_8_Enable
  Decoder_3_to_8_Enable(1) : Decoders_Lib/Decoders_Lib/Decoder_3_to_8_Enable
  Decoder_3_to_8_Enable(2) : Decoders_Lib/Decoders_Lib/Decoder_3_to_8_Enable
  G_Bit(00) : Memory_Blocks_Lib/Memory_Blocks_Lib/G_Bit
  G_Bit(01) : Memory_Blocks_Lib/Memory_Blocks_Lib/G_Bit
  G_Bit(02) : Memory_Blocks_Lib/Memory_Blocks_Lib/G_Bit
  G_Bit(03) : Memory_Blocks_Lib/Memory_Blocks_Lib/G_Bit
  G_Bit(04) : Memory_Blocks_Lib/Memory_Blocks_Lib/G_Bit
  G_Bit(05) : Memory_Blocks_Lib/Memory_Blocks_Lib/G_Bit
  G_Bit(06) : Memory_Blocks_Lib/Memory_Blocks_Lib/G_Bit
  G_Bit(07) : Memory_Blocks_Lib/Memory_Blocks_Lib/G_Bit
  G_Bit(08) : Memory_Blocks_Lib/Memory_Blocks_Lib/G_Bit
  G_Bit(09) : Memory_Blocks_Lib/Memory_Blocks_Lib/G_Bit
  G_Bit(10) : Memory_Blocks_Lib/Memory_Blocks_Lib/G_Bit
  G_Bit(11) : Memory_Blocks_Lib/Memory_Blocks_Lib/G_Bit
  G_Bit(12) : Memory_Blocks_Lib/Memory_Blocks_Lib/G_Bit
  G_Bit(13) : Memory_Blocks_Lib/Memory_Blocks_Lib/G_Bit
  G_Bit(14) : Memory_Blocks_Lib/Memory_Blocks_Lib/G_Bit
  G_Bit(15) : Memory_Blocks_Lib/Memory_Blocks_Lib/G_Bit
  G_Bit(16) : Memory_Blocks_Lib/Memory_Blocks_Lib/G_Bit
  G_Bit(17) : Memory_Blocks_Lib/Memory_Blocks_Lib/G_Bit
  G_Bit(18) : Memory_Blocks_Lib/Memory_Blocks_Lib/G_Bit
  G_Bit(19) : Memory_Blocks_Lib/Memory_Blocks_Lib/G_Bit
  G_Bit(20) : Memory_Blocks_Lib/Memory_Blocks_Lib/G_Bit
  G_Bit(21) : Memory_Blocks_Lib/Memory_Blocks_Lib/G_Bit
  G_Bit(22) : Memory_Blocks_Lib/Memory_Blocks_Lib/G_Bit
  G_Bit(23) : Memory_Blocks_Lib/Memory_Blocks_Lib/G_Bit
  Mux : Mux  Inputs=24
  Terminator{,1..11} (12 alike) : Terminator
  Get_Pixel(1b) : Outport
  Data_Out(24b) : Outport  Port=2
  wires:
  Bus Selector/1 -> Terminator10/1  "<signal1>"
  Bus Selector/2 -> Terminator11/1  "<signal2>"
  Bus Selector/3 -> Terminator7/1  "<signal3>"
  Bus Selector/4 -> Terminator8/1  "<signal4>"
  Bus Selector/5 -> Terminator9/1  "<signal5>"
  Bus Selector/6 -> Terminator4/1  "<signal6>"
  Bus Selector/7 -> Terminator5/1  "<signal7>"
  Bus Selector/8 -> Terminator6/1  "<signal8>"
  Bus Selector/13 -> Decoder_2_to_4/2, Bit_Multiplexer_4_to_1/2  "<signal13>"
  Decoder_3_to_8_Enable(1)/8 -> G_Bit(08)/2
  Bus Selector/11 -> Terminator2/1  "<signal11>"
  Decoder_3_to_8_Enable(1)/6 -> G_Bit(10)/2
  Decoder_3_to_8_Enable(1)/2 -> G_Bit(14)/2
  Decoder_3_to_8_Enable(1)/1 -> G_Bit(15)/2
  Sel_Pos_Y(2B)/1 -> Bus Selector/1
  CLK/1 -> G_Bit(23)/5, G_Bit(22)/5, G_Bit(21)/5, G_Bit(20)/5, G_Bit(19)/5, G_Bit(18)/5, G_Bit(17)/5, G_Bit(16)/5, G_Bit(15)/5, G_Bit(14)/5, G_Bit(13)/5, G_Bit(12)/5, G_Bit(11)/5, G_Bit(10)/5, G_Bit(09)/5, G_Bit(08)/5, G_Bit(07)/5, G_Bit(06)/5, G_Bit(05)/5, G_Bit(04)/5, G_Bit(03)/5, G_Bit(02)/5, G_Bit(01)/5, G_Bit(00)/5
  Decoder_2_to_4/2 -> Decoder_3_to_8_Enable(0)/1
  Decoder_2_to_4/1 -> Terminator3/1
  Bus Selector/15 -> Bit_Multiplexer_8_to_1(1)/2, Bit_Multiplexer_8_to_1(0)/2, Bit_Multiplexer_8_to_1(2)/2, Decoder_3_to_8_Enable(2)/3, Decoder_3_to_8_Enable(1)/3, Decoder_3_to_8_Enable(0)/3  "<signal15>"
  Decoder_2_to_4/3 -> Decoder_3_to_8_Enable(1)/1
  Decoder_3_to_8_Enable(0)/3 -> G_Bit(21)/2
  Decoder_3_to_8_Enable(0)/2 -> G_Bit(22)/2
  Decoder_3_to_8_Enable(1)/3 -> G_Bit(13)/2
  Decoder_3_to_8_Enable(2)/3 -> G_Bit(05)/2
  Decoder_3_to_8_Enable(1)/4 -> G_Bit(12)/2
  Decoder_3_to_8_Enable(1)/7 -> G_Bit(09)/2
  Decoder_3_to_8_Enable(1)/5 -> G_Bit(11)/2
  Decoder_3_to_8_Enable(2)/1 -> G_Bit(07)/2
  Decoder_3_to_8_Enable(2)/8 -> G_Bit(00)/2
  Decoder_3_to_8_Enable(0)/8 -> G_Bit(16)/2
  Decoder_3_to_8_Enable(2)/5 -> G_Bit(03)/2
  Decoder_3_to_8_Enable(2)/7 -> G_Bit(01)/2
  Decoder_3_to_8_Enable(0)/4 -> G_Bit(20)/2
  Decoder_3_to_8_Enable(0)/7 -> G_Bit(17)/2
  Decoder_3_to_8_Enable(2)/2 -> G_Bit(06)/2
  Decoder_3_to_8_Enable(0)/5 -> G_Bit(19)/2
  Decoder_3_to_8_Enable(2)/4 -> G_Bit(04)/2
  Decoder_3_to_8_Enable(0)/6 -> G_Bit(18)/2
  Decoder_3_to_8_Enable(2)/6 -> G_Bit(02)/2
  Decoder_3_to_8_Enable(0)/1 -> G_Bit(23)/2
  Bus Selector/9 -> Terminator/1  "<signal9>"
  Bus Selector/10 -> Terminator1/1  "<signal10>"
  Bus Selector/14 -> Bit_Multiplexer_8_to_1(1)/1, Bit_Multiplexer_8_to_1(0)/1, Bit_Multiplexer_8_to_1(2)/1, Decoder_3_to_8_Enable(2)/2, Decoder_3_to_8_Enable(1)/2, Decoder_3_to_8_Enable(0)/2  "<signal14>"
  Decoder_2_to_4/4 -> Decoder_3_to_8_Enable(2)/1
  Bus Selector/16 -> Decoder_3_to_8_Enable(2)/4, Decoder_3_to_8_Enable(1)/4, Decoder_3_to_8_Enable(0)/4, Bit_Multiplexer_8_to_1(1)/3, Bit_Multiplexer_8_to_1(0)/3, Bit_Multiplexer_8_to_1(2)/3  "<signal16>"
  Bus Selector/12 -> Bit_Multiplexer_4_to_1/1, Decoder_2_to_4/1  "<signal12>"
  Sel_Pos_X(1b)/1 -> G_Bit(01)/1, G_Bit(00)/1, G_Bit(02)/1, G_Bit(03)/1, G_Bit(04)/1, G_Bit(05)/1, G_Bit(06)/1, G_Bit(07)/1, G_Bit(08)/1, G_Bit(09)/1, G_Bit(10)/1, G_Bit(11)/1, G_Bit(12)/1, G_Bit(13)/1, G_Bit(14)/1, G_Bit(15)/1, G_Bit(16)/1, G_Bit(17)/1, G_Bit(18)/1, G_Bit(19)/1, G_Bit(20)/1, G_Bit(21)/1, G_Bit(22)/1, G_Bit(23)/1
  Data_In(1b)/1 -> G_Bit(23)/3, G_Bit(22)/3, G_Bit(21)/3, G_Bit(20)/3, G_Bit(19)/3, G_Bit(18)/3, G_Bit(17)/3, G_Bit(16)/3, G_Bit(15)/3, G_Bit(14)/3, G_Bit(13)/3, G_Bit(12)/3, G_Bit(11)/3, G_Bit(10)/3, G_Bit(09)/3, G_Bit(08)/3, G_Bit(07)/3, G_Bit(06)/3, G_Bit(05)/3, G_Bit(04)/3, G_Bit(03)/3, G_Bit(02)/3, G_Bit(01)/3, G_Bit(00)/3
  G_Bit(23)/1 -> Bit_Multiplexer_8_to_1(0)/4, Mux/1
  G_Bit(22)/1 -> Bit_Multiplexer_8_to_1(0)/5, Mux/2
  G_Bit(21)/1 -> Bit_Multiplexer_8_to_1(0)/6, Mux/3
  G_Bit(20)/1 -> Bit_Multiplexer_8_to_1(0)/7, Mux/4
  G_Bit(19)/1 -> Bit_Multiplexer_8_to_1(0)/8, Mux/5
  G_Bit(18)/1 -> Bit_Multiplexer_8_to_1(0)/9, Mux/6
  G_Bit(17)/1 -> Bit_Multiplexer_8_to_1(0)/10, Mux/7
  G_Bit(15)/1 -> Bit_Multiplexer_8_to_1(1)/4, Mux/9
  G_Bit(14)/1 -> Bit_Multiplexer_8_to_1(1)/5, Mux/10
  G_Bit(13)/1 -> Mux/11, Bit_Multiplexer_8_to_1(1)/6
  G_Bit(12)/1 -> Bit_Multiplexer_8_to_1(1)/7, Mux/12
  G_Bit(11)/1 -> Bit_Multiplexer_8_to_1(1)/8, Mux/13
  G_Bit(10)/1 -> Bit_Multiplexer_8_to_1(1)/9, Mux/14
  G_Bit(09)/1 -> Bit_Multiplexer_8_to_1(1)/10, Mux/15
  G_Bit(08)/1 -> Bit_Multiplexer_8_to_1(1)/11, Mux/16
  G_Bit(07)/1 -> Bit_Multiplexer_8_to_1(2)/4, Mux/17
  G_Bit(06)/1 -> Bit_Multiplexer_8_to_1(2)/5, Mux/18
  G_Bit(05)/1 -> Bit_Multiplexer_8_to_1(2)/6, Mux/19
  G_Bit(04)/1 -> Bit_Multiplexer_8_to_1(2)/7, Mux/20
  G_Bit(03)/1 -> Bit_Multiplexer_8_to_1(2)/8, Mux/21
  G_Bit(02)/1 -> Bit_Multiplexer_8_to_1(2)/9, Mux/22
  G_Bit(01)/1 -> Mux/23, Bit_Multiplexer_8_to_1(2)/10
  G_Bit(00)/1 -> Bit_Multiplexer_8_to_1(2)/11, Mux/24
  Mux/1 -> Bit to Integer Converter/1
  Bit to Integer Converter/1 -> Data_Out(24b)/1
  Write(1b)/1 -> G_Bit(23)/4, G_Bit(22)/4, G_Bit(21)/4, G_Bit(20)/4, G_Bit(19)/4, G_Bit(18)/4, G_Bit(17)/4, G_Bit(16)/4, G_Bit(15)/4, G_Bit(13)/4, G_Bit(12)/4, G_Bit(11)/4, G_Bit(10)/4, G_Bit(09)/4, G_Bit(08)/4, G_Bit(07)/4, G_Bit(06)/4, G_Bit(05)/4, G_Bit(04)/4, G_Bit(03)/4, G_Bit(02)/4, G_Bit(01)/4, G_Bit(00)/4, G_Bit(14)/4
  G_Bit(16)/1 -> Bit_Multiplexer_8_to_1(0)/11, Mux/8
  Bit_Multiplexer_8_to_1(0)/1 -> Bit_Multiplexer_4_to_1/4
  Bit_Multiplexer_8_to_1(1)/1 -> Bit_Multiplexer_4_to_1/5
  Bit_Multiplexer_8_to_1(2)/1 -> Bit_Multiplexer_4_to_1/6
  Constant/1 -> Bit_Multiplexer_4_to_1/3
  Bit_Multiplexer_4_to_1/1 -> Get_Pixel(1b)/1

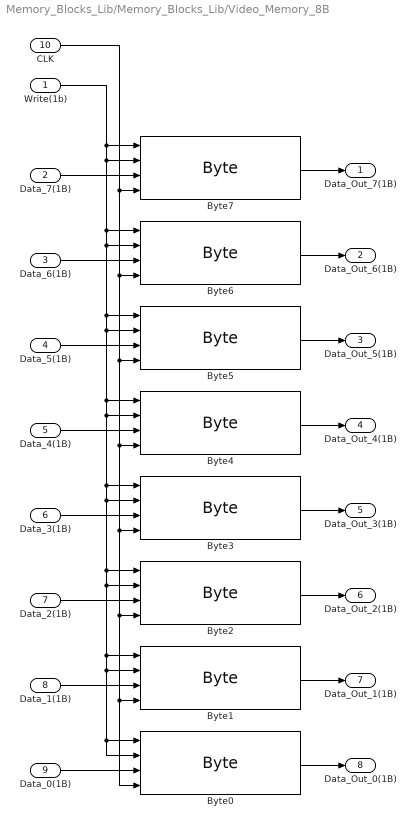
== system Memory_Blocks_Lib/Memory_Blocks_Lib/Video_Memory_8B ==
  Write(1b) : Inport
  Data_7(1B) : Inport  Port=2
  Data_6(1B) : Inport  Port=3
  Data_5(1B) : Inport  Port=4
  Data_4(1B) : Inport  Port=5
  Data_3(1B) : Inport  Port=6
  Data_2(1B) : Inport  Port=7
  Data_1(1B) : Inport  Port=8
  Data_0(1B) : Inport  Port=9
  CLK : Inport  Port=10
  Byte{0..7} (8 alike) : Memory_Blocks_Lib/Memory_Blocks_Lib/Byte
  Data_Out_7(1B) : Outport
  Data_Out_6(1B) : Outport  Port=2
  Data_Out_5(1B) : Outport  Port=3
  Data_Out_4(1B) : Outport  Port=4
  Data_Out_3(1B) : Outport  Port=5
  Data_Out_2(1B) : Outport  Port=6
  Data_Out_1(1B) : Outport  Port=7
  Data_Out_0(1B) : Outport  Port=8
  wires:
  Data_0(1B)/1 -> Byte0/3
  CLK/1 -> Byte0/4, Byte1/4, Byte2/4, Byte3/4, Byte4/4, Byte5/4, Byte6/4, Byte7/4
  Write(1b)/1 -> Byte7/1, Byte7/2, Byte6/1, Byte6/2, Byte5/1, Byte5/2, Byte4/1, Byte4/2, Byte3/1, Byte3/2, Byte2/1, Byte2/2, Byte1/1, Byte1/2, Byte0/1, Byte0/2
  Data_1(1B)/1 -> Byte1/3
  Data_2(1B)/1 -> Byte2/3
  Data_3(1B)/1 -> Byte3/3
  Data_4(1B)/1 -> Byte4/3
  Data_5(1B)/1 -> Byte5/3
  Data_6(1B)/1 -> Byte6/3
  Data_7(1B)/1 -> Byte7/3
  Byte7/1 -> Data_Out_7(1B)/1
  Byte6/1 -> Data_Out_6(1B)/1
  Byte5/1 -> Data_Out_5(1B)/1
  Byte4/1 -> Data_Out_4(1B)/1
  Byte3/1 -> Data_Out_3(1B)/1
  Byte2/1 -> Data_Out_2(1B)/1
  Byte1/1 -> Data_Out_1(1B)/1
  Byte0/1 -> Data_Out_0(1B)/1

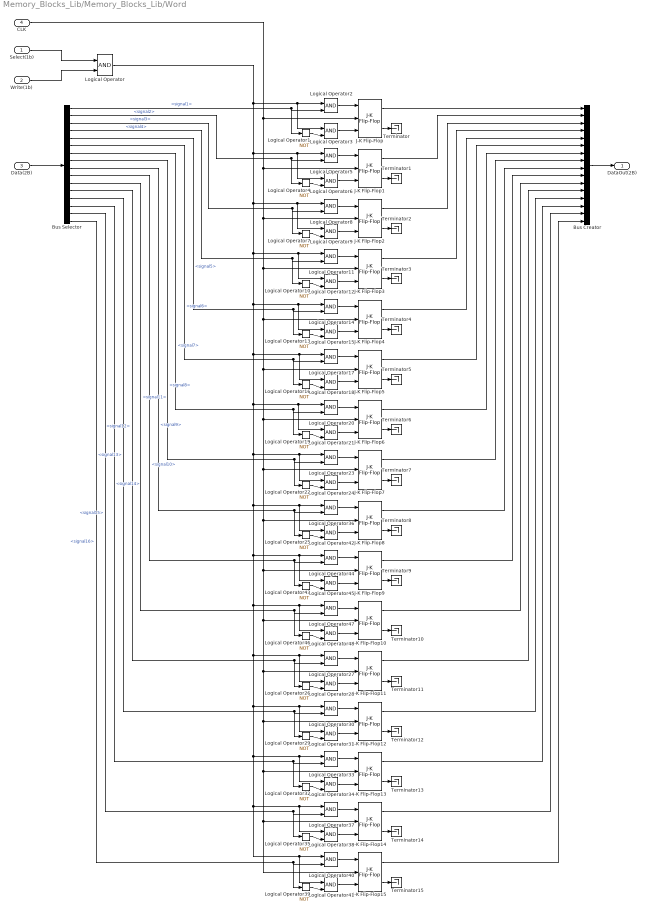
== system Memory_Blocks_Lib/Memory_Blocks_Lib/Word ==
  Select(1b) : Inport
  Write(1b) : Inport  Port=2
  Data(2B) : Inport  Port=3
  CLK : Inport  Port=4  OutDataTypeStr=double
  Bus Creator : BusCreator  Inputs=16
  Bus Selector : BusSelector  OutputSignals=signal1,signal2,signal3,signal4,signal5,signal6,signal7,signal8,signal9,signal10,signal11,signal12,signal13,signal14,signal15,signal16
  J-K Flip-Flop{,1..15} (16 alike) : simulink_extras/Flip Flops/J-K Flip-Flop  initial_condition=0
  Logical Operator{,2..3,5..6,8..9,11..12,14..15,17..18,20..21,23..24,27..28,30..31,33..34,36..38,40..42,44..45,47..48} (33 alike) : Logic  IconShape=distinctive  AllPortsSameDT=off  OutDataTypeStr=boolean
  Logical Operator{1,4,7,10,13,16,19,22,25..26,29,32,35,39,43,46} (16 alike) : Logic  Operator=NOT  IconShape=distinctive  AllPortsSameDT=off  OutDataTypeStr=boolean
  Terminator{,1..15} (16 alike) : Terminator
  DataOut(2B) : Outport
  wires:
  Write(1b)/1 -> Logical Operator/2
  Select(1b)/1 -> Logical Operator/1
  Data(2B)/1 -> Bus Selector/1
  J-K Flip-Flop7/1 -> Bus Creator/8
  J-K Flip-Flop6/1 -> Bus Creator/7
  J-K Flip-Flop5/1 -> Bus Creator/6
  J-K Flip-Flop4/1 -> Bus Creator/5
  J-K Flip-Flop3/1 -> Bus Creator/4
  J-K Flip-Flop2/1 -> Bus Creator/3
  J-K Flip-Flop1/1 -> Bus Creator/2
  J-K Flip-Flop/1 -> Bus Creator/1
  Bus Creator/1 -> DataOut(2B)/1
  Bus Selector/1 -> Logical Operator1/1, Logical Operator2/2  "<signal1>"
  J-K Flip-Flop/2 -> Terminator/1
  Logical Operator1/1 -> Logical Operator3/2
  Logical Operator2/1 -> J-K Flip-Flop/1
  Logical Operator3/1 -> J-K Flip-Flop/3
  Bus Selector/2 -> Logical Operator4/1, Logical Operator5/2  "<signal2>"
  J-K Flip-Flop1/2 -> Terminator1/1
  Logical Operator4/1 -> Logical Operator6/2
  Logical Operator5/1 -> J-K Flip-Flop1/1
  Logical Operator6/1 -> J-K Flip-Flop1/3
  Bus Selector/3 -> Logical Operator7/1, Logical Operator8/2  "<signal3>"
  J-K Flip-Flop2/2 -> Terminator2/1
  Logical Operator7/1 -> Logical Operator9/2
  Logical Operator8/1 -> J-K Flip-Flop2/1
  Logical Operator9/1 -> J-K Flip-Flop2/3
  Bus Selector/4 -> Logical Operator11/2, Logical Operator10/1  "<signal4>"
  J-K Flip-Flop3/2 -> Terminator3/1
  Logical Operator10/1 -> Logical Operator12/2
  Logical Operator11/1 -> J-K Flip-Flop3/1
  Logical Operator12/1 -> J-K Flip-Flop3/3
  Bus Selector/5 -> Logical Operator13/1, Logical Operator14/2  "<signal5>"
  J-K Flip-Flop4/2 -> Terminator4/1
  Logical Operator13/1 -> Logical Operator15/2
  Logical Operator14/1 -> J-K Flip-Flop4/1
  Logical Operator15/1 -> J-K Flip-Flop4/3
  Bus Selector/6 -> Logical Operator16/1, Logical Operator17/2  "<signal6>"
  J-K Flip-Flop5/2 -> Terminator5/1
  Logical Operator16/1 -> Logical Operator18/2
  Logical Operator17/1 -> J-K Flip-Flop5/1
  Logical Operator18/1 -> J-K Flip-Flop5/3
  Bus Selector/7 -> Logical Operator19/1, Logical Operator20/2  "<signal7>"
  J-K Flip-Flop6/2 -> Terminator6/1
  Logical Operator19/1 -> Logical Operator21/2
  Logical Operator20/1 -> J-K Flip-Flop6/1
  Logical Operator21/1 -> J-K Flip-Flop6/3
  Bus Selector/8 -> Logical Operator22/1, Logical Operator23/2  "<signal8>"
  J-K Flip-Flop7/2 -> Terminator7/1
  Logical Operator22/1 -> Logical Operator24/2
  Logical Operator23/1 -> J-K Flip-Flop7/1
  Logical Operator24/1 -> J-K Flip-Flop7/3
  J-K Flip-Flop15/1 -> Bus Creator/16
  J-K Flip-Flop14/1 -> Bus Creator/15
  J-K Flip-Flop13/1 -> Bus Creator/14
  J-K Flip-Flop12/1 -> Bus Creator/13
  J-K Flip-Flop11/1 -> Bus Creator/12
  J-K Flip-Flop10/1 -> Bus Creator/11
  J-K Flip-Flop9/1 -> Bus Creator/10
  J-K Flip-Flop8/1 -> Bus Creator/9
  Bus Selector/9 -> Logical Operator25/1, Logical Operator36/2  "<signal9>"
  J-K Flip-Flop8/2 -> Terminator8/1
  Logical Operator25/1 -> Logical Operator42/2
  Logical Operator36/1 -> J-K Flip-Flop8/1
  Logical Operator42/1 -> J-K Flip-Flop8/3
  Bus Selector/10 -> Logical Operator43/1, Logical Operator44/2  "<signal10>"
  J-K Flip-Flop9/2 -> Terminator9/1
  Logical Operator43/1 -> Logical Operator45/2
  Logical Operator44/1 -> J-K Flip-Flop9/1
  Logical Operator45/1 -> J-K Flip-Flop9/3
  Bus Selector/11 -> Logical Operator46/1, Logical Operator47/2  "<signal11>"
  J-K Flip-Flop10/2 -> Terminator10/1
  Logical Operator46/1 -> Logical Operator48/2
  Logical Operator47/1 -> J-K Flip-Flop10/1
  Logical Operator48/1 -> J-K Flip-Flop10/3
  Bus Selector/12 -> Logical Operator27/2, Logical Operator26/1  "<signal12>"
  J-K Flip-Flop11/2 -> Terminator11/1
  Logical Operator26/1 -> Logical Operator28/2
  Logical Operator27/1 -> J-K Flip-Flop11/1
  Logical Operator28/1 -> J-K Flip-Flop11/3
  Bus Selector/13 -> Logical Operator30/2, Logical Operator29/1  "<signal13>"
  J-K Flip-Flop12/2 -> Terminator12/1
  Logical Operator29/1 -> Logical Operator31/2
  Logical Operator30/1 -> J-K Flip-Flop12/1
  Logical Operator31/1 -> J-K Flip-Flop12/3
  Bus Selector/14 -> Logical Operator33/2, Logical Operator32/1  "<signal14>"
  J-K Flip-Flop13/2 -> Terminator13/1
  Logical Operator32/1 -> Logical Operator34/2
  Logical Operator33/1 -> J-K Flip-Flop13/1
  Logical Operator34/1 -> J-K Flip-Flop13/3
  Bus Selector/15 -> Logical Operator35/1, Logical Operator37/2  "<signal15>"
  J-K Flip-Flop14/2 -> Terminator14/1
  Logical Operator35/1 -> Logical Operator38/2
  Logical Operator37/1 -> J-K Flip-Flop14/1
  Logical Operator38/1 -> J-K Flip-Flop14/3
  Bus Selector/16 -> Logical Operator39/1, Logical Operator40/2  "<signal16>"
  J-K Flip-Flop15/2 -> Terminator15/1
  CLK/1 -> J-K Flip-Flop/2, J-K Flip-Flop1/2, J-K Flip-Flop2/2, J-K Flip-Flop3/2, J-K Flip-Flop6/2, J-K Flip-Flop7/2, J-K Flip-Flop8/2, J-K Flip-Flop9/2, J-K Flip-Flop10/2, J-K Flip-Flop11/2, J-K Flip-Flop12/2, J-K Flip-Flop15/2, J-K Flip-Flop14/2, J-K Flip-Flop13/2, J-K Flip-Flop5/2, J-K Flip-Flop4/2
  Logical Operator/1 -> Logical Operator3/1, Logical Operator2/1, Logical Operator6/1, Logical Operator5/1, Logical Operator9/1, Logical Operator8/1, Logical Operator12/1, Logical Operator11/1, Logical Operator15/1, Logical Operator14/1, Logical Operator18/1, Logical Operator17/1, Logical Operator21/1, Logical Operator20/1, Logical Operator24/1, Logical Operator23/1, Logical Operator42/1, Logical Operator36/1, Logical Operator45/1, Logical Operator44/1, Logical Operator48/1, Logical Operator47/1, Logical Operator28/1, Logical Operator27/1, Logical Operator31/1, Logical Operator30/1, Logical Operator34/1, Logical Operator33/1, Logical Operator38/1, Logical Operator37/1, Logical Operator41/1, Logical Operator40/1
  Logical Operator39/1 -> Logical Operator41/2
  Logical Operator40/1 -> J-K Flip-Flop15/1
  Logical Operator41/1 -> J-K Flip-Flop15/3
